simulink model "rpitest"  (R2024b)
settings: Solver=FixedStepAuto  StartTime=0.0  StopTime=inf  FixedStep=1/4000  RelTol=1e-3  EnableMultiTasking=on
libraries: raspberrypiCommlib x5, stmutilitieslib x2, simulink x1
settings Model: ExtModeTrigDuration=2  Creator=u0130154  LastModifiedBy=u0130154
settings SolverCC: PositivePriorityOrder=on  AutoInsertRateTranBlk=on
settings OptimizationCC: EnhancedBackFolding=on  PassReuseOutputArgsAs=Individual arguments  ZeroExternalMemoryAtStartup=off  ZeroInternalMemoryAtStartup=off  MaxStackSize=200000  OptimizeBlockOrder=speed  DifferentSizesBufferReuse=on  OptimizationCustomize=off  EfficientTunableParamExpr=on
settings DebuggingCC: ParameterTunabilityLossMsg=error
settings HardwareCC: ProdBitPerLong=64  ProdLargestAtomicInteger=LongLong  ProdLargestAtomicFloat=Double  ProdLongLongMode=on  ProdHWDeviceType=ARM Compatible->ARM Cortex-A (64-bit)
settings RTWCC: Description=Embedded Coder  SystemTargetFile=ert.tlc  HardwareBoard=Raspberry Pi (64bit)  TLCOptions="-aInlineSetEventsForThisBaseRateFcn=TLC_FALSE -aSuppressMultiTaskScheduler=TLC_FALSE  -aRateBasedStepFcn=0"  TemplateMakefile=ert_default_tmf  Toolchain=GNU GCC Embedded Linux  BuildConfiguration=Faster Runs
settings CodeAppCC: ForceParamTrailComments=on  IgnoreCustomStorageClasses=off  OperatorAnnotations=on  SimulinkDataObjDesc=on  SFDataObjDesc=on  InsertBlockDesc=on
settings ERTTargetCC: CodeReplacementLibrary=ARM Cortex-A CMSIS  SupportVariableSizeSignals=on  ExtModeTransport=2  ExtModeStaticAlloc=on  ExtModeMexFile=ext_xcp  ExtModeIntrfLevel=Level2 - Open  InlinedParameterPlacement=Hierarchical

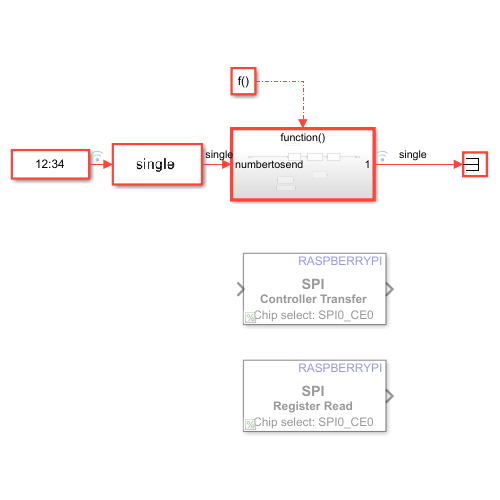
[thumbnail: Simulink's stored preview of the top-level diagram]
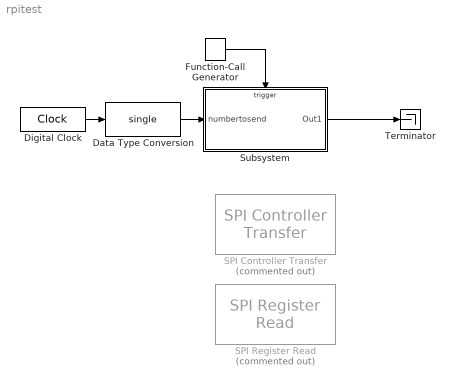
== system rpitest ==
  Data Type Conversion : DataTypeConversion  OutDataTypeStr=single  SaturateOnIntegerOverflow=off  RndMeth=Floor
  Digital Clock : DigitalClock  SampleTime=-1
  Function-Call Generator : simulink/Ports & Subsystems/Function-Call Generator  sample_time=1/4000  numberOfIterations=1  DisallowWideOutput=off
  SPI Controller Transfer : raspberrypiCommlib/SPI Controller Transfer  Commented=on  BoardProperty=Pi 4 Model B  SSPin=SPI0_CE0  SPIModule=uint32(0)  Mode=Master  BusSpeed=1000000  Pin=uint32(0)  FirstBitToTransfer=Most significant bit (MSB)  ClockMode=0  BlockFunction=Transfer  RegisterAddress=0  OutputDataType=int8  OutputDataLength=1
  SPI Register Read : raspberrypiCommlib/SPI Register Read  Commented=on  BoardProperty=Pi 2 Model B  SSPin=SPI0_CE0  SPIModule=uint32(0)  Mode=Master  BusSpeed=1000000  Pin=uint32(0)  FirstBitToTransfer=Most significant bit (MSB)  ClockMode=0  BlockFunction=Read  RegisterAddress=0  OutputDataType=int8  OutputDataLength=1  SampleTime=0.1
  Subsystem : Subsystem
  Terminator : Terminator
  wires:
  Digital Clock/1 -> Data Type Conversion/1
  Function-Call Generator/1 -> Subsystem/Trigger
  Data Type Conversion/1 -> Subsystem/1(numbertosend)
  Subsystem/1(Out1) -> Terminator/1

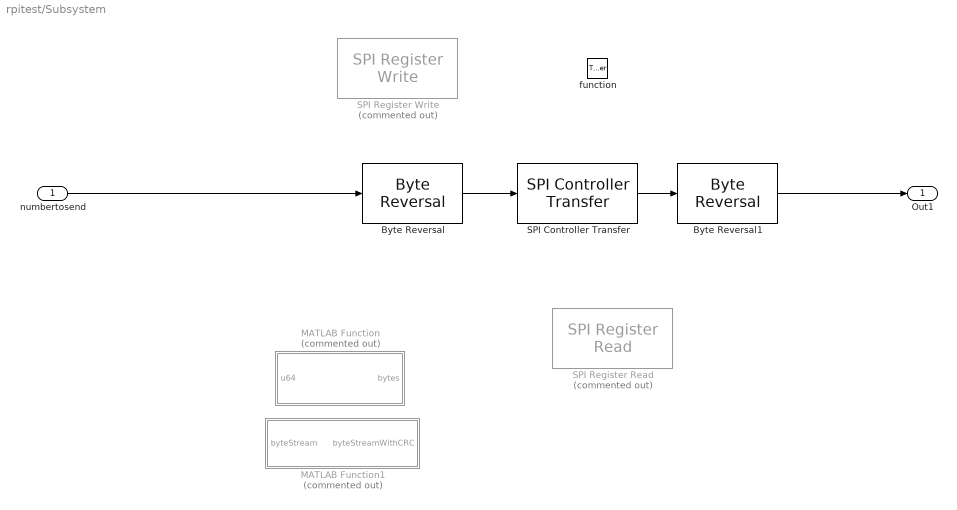
== system rpitest/Subsystem ==
  numbertosend : Inport
  function : TriggerPort  TriggerType=function-call  VariantControl=(inherit)
  Byte Reversal : stmutilitieslib/Byte Reversal  numInp=1  blockPlatform=stm32f4discovery
  Byte Reversal1 : stmutilitieslib/Byte Reversal  numInp=1  blockPlatform=stm32f4discovery
  MATLAB Function : MATLAB Function  Commented=on  TreatAsAtomicUnit=on
  MATLAB Function1 : MATLAB Function  Commented=on  TreatAsAtomicUnit=on
  SPI Controller Transfer : raspberrypiCommlib/SPI Controller Transfer  BoardProperty=Pi 4 Model B  SSPin=SPI0_CE0  SPIModule=uint32(0)  Mode=Master  BusSpeed=1000000  Pin=uint32(0)  FirstBitToTransfer=Most significant bit (MSB)  ClockMode=0  BlockFunction=Transfer  RegisterAddress=0  OutputDataType=int8  OutputDataLength=1
  SPI Register Read : raspberrypiCommlib/SPI Register Read  Commented=on  BoardProperty=Pi 2 Model B  SSPin=SPI0_CE0  SPIModule=uint32(0)  Mode=Master  BusSpeed=1000000  Pin=uint32(0)  FirstBitToTransfer=Most significant bit (MSB)  ClockMode=0  BlockFunction=Read  RegisterAddress=0  OutputDataType=int8  OutputDataLength=1  SampleTime=0.1
  SPI Register Write : raspberrypiCommlib/SPI Register Write  Commented=on  BoardProperty=Pi 4 Model B  SSPin=SPI0_CE0  SPIModule=uint32(0)  Mode=Master  BusSpeed=1000000  Pin=uint32(0)  FirstBitToTransfer=Most significant bit (MSB)  ClockMode=0  BlockFunction=Write  RegisterAddress=0xFF  OutputDataType=int8  OutputDataLength=1
  Out1 : Outport
  wires:
  SPI Controller Transfer/1 -> Byte Reversal1/1
  numbertosend/1 -> Byte Reversal/1
  Byte Reversal/1 -> SPI Controller Transfer/1
  Byte Reversal1/1 -> Out1/1

== matlab function rpitest/Subsystem/MATLAB Function ==
  data: u64 input; bytes output
function bytes = splitUint64ToBytes(u64)
    % Ensure input is uint64
    if ~isa(u64, 'uint64')
        error('Input must be a uint64 value.');
    end
    
    % Preallocate array for the 8 bytes
    bytes = uint8(zeros(1, 8));
    
    % Extract each byte by shifting and masking
    bytes(1) = uint8(bitand(u64, uint64(0xFF)));          % Byte 1 (LSB)
    bytes(2) = uint8(bitand(bitshift(u64, -8), uint64(0xFF))); % Byte 2
    bytes(3) = uint8(bitand(bitshift(u64, -16), uint64(0xFF))); % Byte 3
    bytes(4) = uint8(bitand(bitshift(u64, -24), uint64(0xFF))); % Byte 4
    bytes(5) = uint8(bitand(bitshift(u64, -32), uint64(0xFF))); % Byte 5
    bytes(6) = uint8(bitand(bitshift(u64, -40), uint64(0xFF))); % Byte 6
    bytes(7) = uint8(bitand(bitshift(u64, -48), uint64(0xFF))); % Byte 7
    bytes(8) = uint8(bitand(bitshift(u64, -56), uint64(0xFF))); % Byte 8 (MSB)
end

== matlab function rpitest/Subsystem/MATLAB Function1 ==
  data: byteStream input uint8; byteStreamWithCRC output uint8
function byteStreamWithCRC = appendCRC(byteStream)
    % AppendCRC - Calculates the CRC (z^8 + z^2 + z + 1) of a byte stream
    % Input: byteStream - vector of uint8 values representing the bytestream
    % Output: byteStreamWithCRC - byteStream with 8-bit CRC appended

    % Define the CRC polynomial coefficients for z^8 + z^2 + z + 1
    polynomial = uint8([1 0 0 1 0 1 1 1]); % Represents x^8 + x^2 + x + 1
    
    % Initialize the CRC register
    crc = uint8(0);
    
    % Process each byte in the byteStream
    for i = 1:numel(byteStream)
        crc = bitxor(crc, byteStream(i)); % XOR with current byte
        % Process each bit of the byte
        for j = 0:7
            % Check if the most significant bit is set
            if bitand(crc, uint8(128)) % 128 = 2^7
                crc = bitshift(crc, -1); % Shift right
                crc = bitxor(crc, uint8(bi2de(polynomial))); % XOR with polynomial
            else
                crc = bitshift(crc, -1); % Shift right
            end
        end
    end
    
    % Append the CRC to the byte stream
    byteStreamWithCRC = [byteStream(:); crc];
end
